simulink model "ControllerTuneLianxi"  (Simulink 9.1)
settings: Solver=VariableStepAuto  StartTime=0.0  StopTime=10  RelTol=1e-3
PreLoadFcn:
  | clear
  | A=[-0.0313 4.4879 0 -9.8; ...
  |    -0.0058 -0.7458 0.9480 0; ...
  |    -0.0002 -0.4479 -0.4609 0; ...
  |    0 0 1 0];
  | B = [0.2063 -0.0516 -0.6532 0; ...
  |      3.4847 -0.0561 0.0193 0]';
  | C = eye(4);
  | D = [0 0 0 0; 0 0 0 0]';
  | Ktheta = 0;
  | KthetaI = 0;
  | KthetaD = 0;
  | Kq = 0;
  | KthetaV = 0;
  | KqV = 0;
  | KDeltaV = 0;
  | Ltheta = 0;
  | Lq = 0;
  | LV = 0;
  | LVI = 0;
  | LVdot = 0;
libraries: simulink x7, checkpacklib x2
settings Model: Creator=McQueen_Zero  LastModifiedBy=McQueen_Zero
settings DataIOCC: SaveFormat=Dataset
settings OptimizationCC: LifeSpan=auto
settings DebuggingCC: UnderspecifiedInitializationDetection=Simplified  MergeDetectMultiDrivingBlocksExec=error  SFUnexpectedBacktrackingDiag=error  SFNoUnconditionalDefaultTransitionDiag=error  SFExecutionAtInitializationDiag=warning
settings HardwareCC: ProdBitPerPointer=64  ProdBitPerSizeT=64  ProdBitPerPtrDiffT=64  ProdLargestAtomicFloat=Float  ProdIntDivRoundTo=Zero  ProdEndianess=LittleEndian  ProdWordSize=64  ProdHWDeviceType=Intel->x86-64 (Windows64)
settings ModelReferenceCC: PropagateSignalLabelsOutOfModel=on
settings CodeAppCC: StateflowObjectComments=off
settings GRTTargetCC: TargetLangStandard=C99 (ISO)  CombineOutputUpdateFcns=on  GRTInterface=off
settings ConfigComp: CovMetricSettings=dwe  CovHtmlReporting=off  CovSaveCumulativeToWorkspaceVar=off  CovSaveSingleToWorkspaceVar=off  CovExternalEMLEnable=on

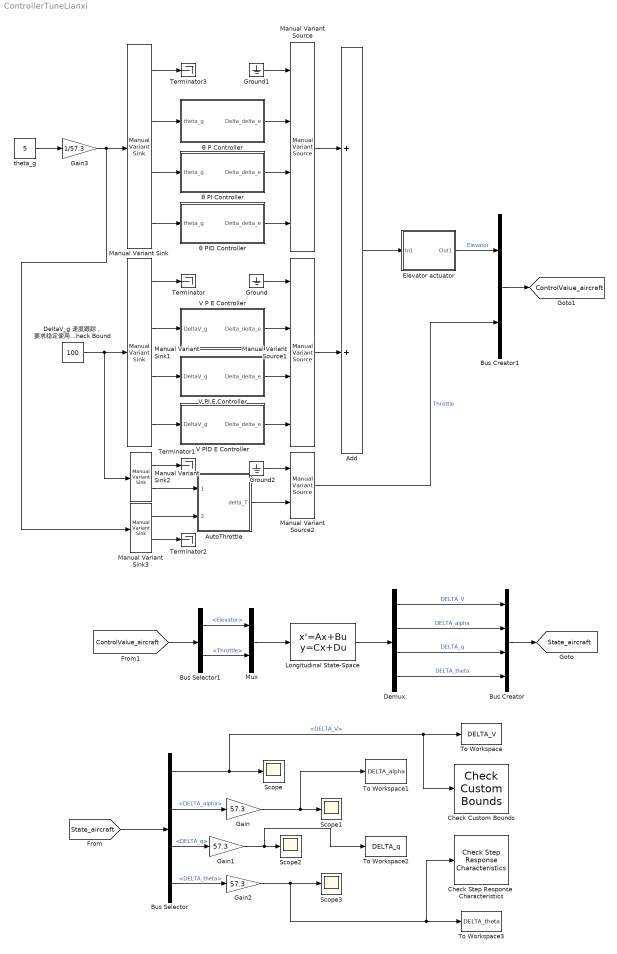
== system ControllerTuneLianxi ==
  Add : Sum
  AutoThrottle : Subsystem  mask{KthetaV=KthetaV, KqV=KqV, KDeltaV=KDeltaV}
      mask prompts: KthetaV "俯仰角增量比例系数"; KqV "俯仰角速率比例系数"; KDeltaV "速度增量比例系数"
  Bus Creator : BusCreator  Inputs=4
  Bus Creator1 : BusCreator  Inputs=2
  Bus Selector : BusSelector  OutputSignals=DELTA_V,DELTA_alpha,DELTA_q,DELTA_theta
  Bus Selector1 : BusSelector  OutputSignals=Elevator,Throttle
  Check Custom Bounds : checkpacklib/Check Custom Bounds  InstantiateOnLoad=on  enabled=on  stopWhenAssertionFail=off  export=off  ViewDlgPos=[]  OpenViewOnLoad=off  LaunchViewOnOpen=off  TimeUnits=seconds  EnableUpperBound=on  UpperBoundTimes=[0 10]  UpperBoundAmplitudes=[1 1]  EnableLowerBound=on  LowerBoundTimes=[0 10]  LowerBoundAmplitudes=[-1 -1]
  Check Step Response  Characteristics : checkpacklib/Check Step Response  Characteristics  InstantiateOnLoad=on  enabled=on  stopWhenAssertionFail=off  export=off  ViewDlgPos=[]  OpenViewOnLoad=off  LaunchViewOnOpen=off  TimeUnits=seconds  EnableStepResponseBound=on  InitialValue=0  FinalValue=5  StepTime=0  RiseTime=2  PercentRise=20  SettlingTime=3  PercentSettling=1  PercentOvershoot=5  PercentUndershoot=1
  "DeltaV_g 速度跟踪， 要求稳定使用 Check Bound " : Constant  Value=100
  Demux : Demux
  Elevator actuator : Subsystem
  Gain : Gain  Gain=57.3
  Gain1 : Gain  Gain=57.3
  Gain2 : Gain  Gain=57.3
  Gain3 : Gain  Gain=1/57.3
  Ground : Ground
  Ground1 : Ground
  Ground2 : Ground
  Longitudinal State-Space : StateSpace  A=A  B=B  C=C  D=D  InitialCondition=0
  Manual Variant Sink : simulink/Signal Routing/Manual Variant Sink  NumChoices=4  OverrideUsingVariant=V_3
      settings: SourceProductName=Simulink
  Manual Variant Sink1 : simulink/Signal Routing/Manual Variant Sink  NumChoices=4  OverrideUsingVariant=V_1
      settings: SourceProductName=Simulink
  Manual Variant Sink2 : simulink/Signal Routing/Manual Variant Sink  NumChoices=2  OverrideUsingVariant=V_1
      settings: SourceProductName=Simulink
  Manual Variant Sink3 : simulink/Signal Routing/Manual Variant Sink  NumChoices=2  OverrideUsingVariant=V_1
      settings: SourceProductName=Simulink
  Manual Variant Source : simulink/Signal Routing/Manual Variant Source  NumChoices=4  OverrideUsingVariant=V_3
      settings: SourceProductName=Simulink
  Manual Variant Source1 : simulink/Signal Routing/Manual Variant Source  NumChoices=4  OverrideUsingVariant=V_1
      settings: SourceProductName=Simulink
  Manual Variant Source2 : simulink/Signal Routing/Manual Variant Source  NumChoices=2  OverrideUsingVariant=V_2
      settings: SourceProductName=Simulink
  Mux : Mux  Inputs=2
  Scope{,1..3} (4 alike) : Scope
  Terminator{,1..3} (4 alike) : Terminator
  To Workspace : ToWorkspace  VariableName=DELTA_V  SaveFormat=Timeseries  SampleTime=-1
  To Workspace1 : ToWorkspace  VariableName=DELTA_alpha  SaveFormat=Timeseries  SampleTime=-1
  To Workspace2 : ToWorkspace  VariableName=DELTA_q  SaveFormat=Timeseries  SampleTime=-1
  To Workspace3 : ToWorkspace  VariableName=DELTA_theta  SaveFormat=Timeseries  SampleTime=-1
  V P E Controller : Subsystem  mask{LV=LV, Ltheta=Ltheta, Lq=Lq}
      mask prompts: LV "速度系数"; Ltheta "俯仰角系数"; Lq "俯仰角速率系数"
  V PI E Controller : Subsystem  mask{LV=LV, LVI=LVI, Ltheta=Ltheta, Lq=Lq}
      mask prompts: LV "速度系数"; LVI "速度积分系数"; Ltheta "俯仰角系数"; Lq "俯仰角速率系数"
  V PID E Controller : Subsystem  mask{LV=LV, LVI=LVI, LVdot=LVdot, Ltheta=Ltheta, Lq=Lq}
      mask prompts: LV "速度系数"; LVI "速度积分系数"; LVdot "速度微分系数"; Ltheta "俯仰角系数"; Lq "俯仰角速率系数"
  theta_g : Constant  Value=5
  θ P Controller : Subsystem  mask{Ktheta=Ktheta, Kq=Kq}
      mask prompts: Ktheta "俯仰角比例系数"; Kq "俯仰角速率比例系数"
  θ PI Controller : Subsystem  mask{Ktheta=Ktheta, KthetaI=KthetaI, Kq=Kq}
      mask prompts: Ktheta "俯仰角比例系数"; KthetaI "俯仰角积分系数"; Kq "俯仰角速率比例系数"
  θ PID Controller : Subsystem  mask{Ktheta=Ktheta, KthetaI=KthetaI, KthetaD=KthetaD, Kq=Kq}
      mask prompts: Ktheta "俯仰角比例系数"; KthetaI "俯仰角积分系数"; KthetaD "俯仰角微分系数"; Kq "俯仰角速率比例系数"
  tag scope: ControlValue_aircraft=global, State_aircraft=global
  wires:
  Demux/3 -> Bus Creator/3  "DELTA_q"
  Gain1/1 -> To Workspace2/1, Scope2/1
  Bus Selector/4 -> Gain2/1  "<DELTA_theta>"
  Bus Selector/2 -> Gain/1  "<DELTA_alpha>"
  Bus Selector/3 -> Gain1/1  "<DELTA_q>"
  [State_aircraft] -> Bus Selector/1
  Demux/2 -> Bus Creator/2  "DELTA_alpha"
  Demux/4 -> Bus Creator/4  "DELTA_theta"
  Demux/1 -> Bus Creator/1  "DELTA_V"
  Gain/1 -> To Workspace1/1, Scope1/1
  Mux/1 -> Longitudinal State-Space/1
  Longitudinal State-Space/1 -> Demux/1
  Bus Creator/1 -> [State_aircraft]
  Gain2/1 -> Check Step Response  Characteristics/1, To Workspace3/1, Scope3/1
  Bus Selector/1 -> Check Custom Bounds/1, To Workspace/1, Scope/1  "<DELTA_V>"
  Bus Selector1/2 -> Mux/2  "<Throttle>"
  Bus Selector1/1 -> Mux/1  "<Elevator>"
  [ControlValue_aircraft] -> Bus Selector1/1
  Elevator actuator/1(Out1) -> Bus Creator1/1  "Elevator"
  Bus Creator1/1 -> [ControlValue_aircraft]
  theta_g/1 -> Gain3/1
  θ P Controller/1(Delta_delta_e) -> Manual Variant Source/2
  θ PI Controller/1(Delta_delta_e) -> Manual Variant Source/3
  θ PID Controller/1(Delta_delta_e) -> Manual Variant Source/4
  Manual Variant Sink/2 -> θ P Controller/1(theta_g)
  Manual Variant Sink/3 -> θ PI Controller/1(theta_g)
  Manual Variant Sink/4 -> θ PID Controller/1(theta_g)
  Gain3/1 -> Manual Variant Sink3/1, Manual Variant Sink/1
  Add/1 -> Elevator actuator/1(In1)
  Manual Variant Source/1 -> Add/1
  V P E Controller/1(Delta_delta_e) -> Manual Variant Source1/2
  Manual Variant Source1/1 -> Add/2
  Ground/1 -> Manual Variant Source1/1
  "DeltaV_g 速度跟踪， 要求稳定使用 Check Bound "/1 -> Manual Variant Sink2/1, Manual Variant Sink1/1
  Manual Variant Sink1/2 -> V P E Controller/1(DeltaV_g)
  Manual Variant Sink1/3 -> V PI E Controller/1(DeltaV_g)
  Manual Variant Sink1/4 -> V PID E Controller/1(DeltaV_g)
  V PI E Controller/1(Delta_delta_e) -> Manual Variant Source1/3
  V PID E Controller/1(Delta_delta_e) -> Manual Variant Source1/4
  Manual Variant Sink1/1 -> Terminator/1
  Manual Variant Sink2/1 -> Terminator1/1
  Manual Variant Sink3/2 -> Terminator2/1
  Manual Variant Sink2/2 -> AutoThrottle/1(DeltaV_g)
  Manual Variant Sink3/1 -> AutoThrottle/2(theta_g)
  Manual Variant Sink/1 -> Terminator3/1
  Ground1/1 -> Manual Variant Source/1
  AutoThrottle/1(delta_T) -> Manual Variant Source2/2
  Ground2/1 -> Manual Variant Source2/1
  Manual Variant Source2/1 -> Bus Creator1/2  "Throttle"

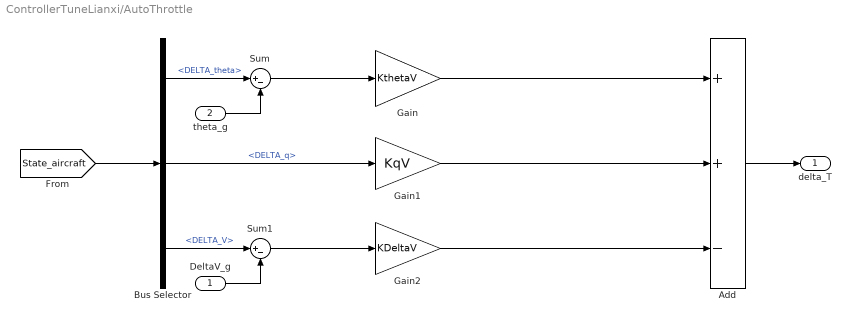
== system ControllerTuneLianxi/AutoThrottle ==
  DeltaV_g : Inport
  theta_g : Inport  Port=2
  Add : Sum  Inputs=++-
  Bus Selector : BusSelector  OutputSignals=DELTA_theta,DELTA_q,DELTA_V
  Gain : Gain  Gain=KthetaV
  Gain1 : Gain  Gain=KqV
  Gain2 : Gain  Gain=KDeltaV
  Sum : Sum  Inputs=|+-
  Sum1 : Sum  Inputs=|+-
  delta_T : Outport
  wires:
  [State_aircraft] -> Bus Selector/1
  Add/1 -> delta_T/1
  Gain1/1 -> Add/2
  Gain/1 -> Add/1
  Bus Selector/2 -> Gain1/1  "<DELTA_q>"
  Bus Selector/1 -> Sum/1  "<DELTA_theta>"
  Bus Selector/3 -> Sum1/1  "<DELTA_V>"
  Sum/1 -> Gain/1
  theta_g/1 -> Sum/2
  Sum1/1 -> Gain2/1
  DeltaV_g/1 -> Sum1/2
  Gain2/1 -> Add/3

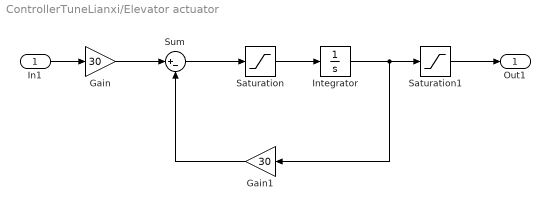
== system ControllerTuneLianxi/Elevator actuator ==
  In1 : Inport
  Gain : Gain  Gain=30
  Gain1 : Gain  Gain=30
  Integrator : Integrator
  Saturation : Saturate  UpperLimit=180  LowerLimit=-180
  Saturation1 : Saturate  UpperLimit=30  LowerLimit=-30
  Sum : Sum  Inputs=|+-
  Out1 : Outport
  wires:
  Saturation/1 -> Integrator/1
  Saturation1/1 -> Out1/1
  In1/1 -> Gain/1
  Gain/1 -> Sum/1
  Sum/1 -> Saturation/1
  Gain1/1 -> Sum/2
  Integrator/1 -> Gain1/1, Saturation1/1

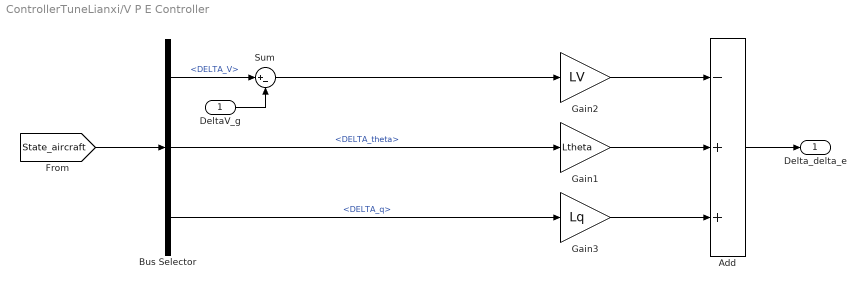
== system ControllerTuneLianxi/V P E Controller ==
  DeltaV_g : Inport
  Add : Sum  Inputs=-++
  Bus Selector : BusSelector  OutputSignals=DELTA_V,DELTA_theta,DELTA_q
  Gain1 : Gain  Gain=Ltheta
  Gain2 : Gain  Gain=LV
  Gain3 : Gain  Gain=Lq
  Sum : Sum  Inputs=|+-
  Delta_delta_e : Outport
  wires:
  [State_aircraft] -> Bus Selector/1
  DeltaV_g/1 -> Sum/2
  Bus Selector/1 -> Sum/1  "<DELTA_V>"
  Sum/1 -> Gain2/1
  Add/1 -> Delta_delta_e/1
  Gain2/1 -> Add/1
  Gain1/1 -> Add/2
  Gain3/1 -> Add/3
  Bus Selector/3 -> Gain3/1  "<DELTA_q>"
  Bus Selector/2 -> Gain1/1  "<DELTA_theta>"

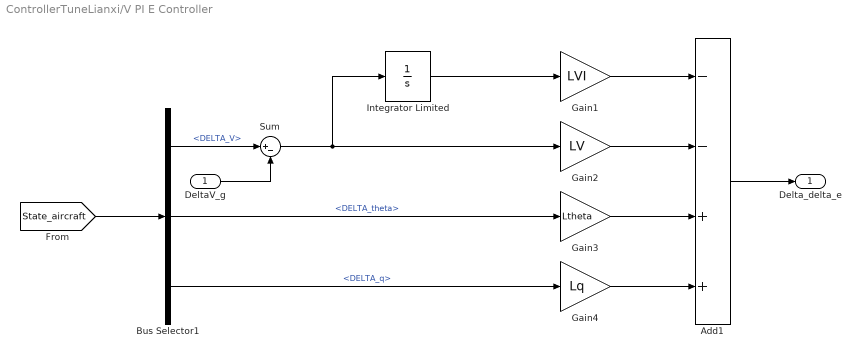
== system ControllerTuneLianxi/V PI E Controller ==
  DeltaV_g : Inport
  Add1 : Sum  Inputs=--++
  Bus Selector1 : BusSelector  OutputSignals=DELTA_V,DELTA_theta,DELTA_q
  Gain1 : Gain  Gain=LVI
  Gain2 : Gain  Gain=LV
  Gain3 : Gain  Gain=Ltheta
  Gain4 : Gain  Gain=Lq
  Integrator Limited : Integrator  LimitOutput=on  UpperSaturationLimit=30/57.3  LowerSaturationLimit=0
  Sum : Sum  Inputs=|+-
  Delta_delta_e : Outport
  wires:
  Add1/1 -> Delta_delta_e/1
  [State_aircraft] -> Bus Selector1/1
  DeltaV_g/1 -> Sum/2
  Bus Selector1/1 -> Sum/1  "<DELTA_V>"
  Gain2/1 -> Add1/2
  Sum/1 -> Integrator Limited/1, Gain2/1
  Gain1/1 -> Add1/1
  Integrator Limited/1 -> Gain1/1
  Gain3/1 -> Add1/3
  Gain4/1 -> Add1/4
  Bus Selector1/3 -> Gain4/1  "<DELTA_q>"
  Bus Selector1/2 -> Gain3/1  "<DELTA_theta>"

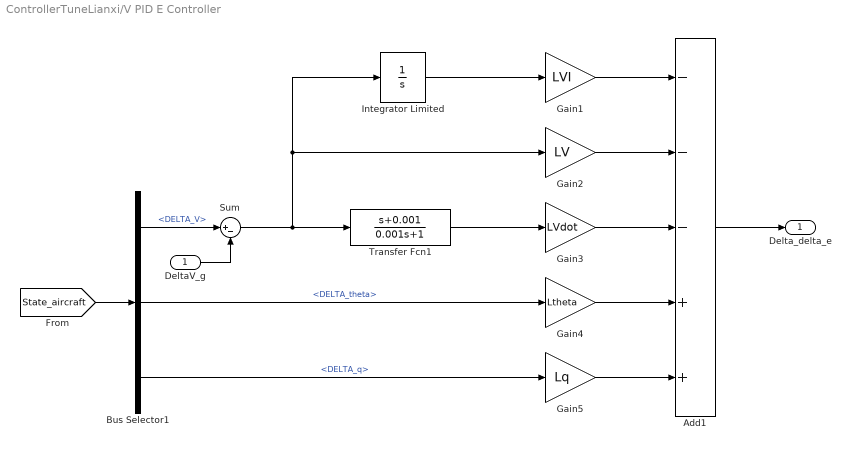
== system ControllerTuneLianxi/V PID E Controller ==
  DeltaV_g : Inport
  Add1 : Sum  Inputs=---++
  Bus Selector1 : BusSelector  OutputSignals=DELTA_V,DELTA_theta,DELTA_q
  Gain1 : Gain  Gain=LVI
  Gain2 : Gain  Gain=LV
  Gain3 : Gain  Gain=LVdot
  Gain4 : Gain  Gain=Ltheta
  Gain5 : Gain  Gain=Lq
  Integrator Limited : Integrator  LimitOutput=on  UpperSaturationLimit=30/57.3  LowerSaturationLimit=0
  Sum : Sum  Inputs=|+-
  Transfer Fcn1 : TransferFcn  Numerator=[1 0.001]  Denominator=[0.001 1]
  Delta_delta_e : Outport
  wires:
  Add1/1 -> Delta_delta_e/1
  [State_aircraft] -> Bus Selector1/1
  DeltaV_g/1 -> Sum/2
  Bus Selector1/1 -> Sum/1  "<DELTA_V>"
  Transfer Fcn1/1 -> Gain3/1
  Gain3/1 -> Add1/3
  Gain2/1 -> Add1/2
  Sum/1 -> Integrator Limited/1, Gain2/1, Transfer Fcn1/1
  Gain1/1 -> Add1/1
  Integrator Limited/1 -> Gain1/1
  Gain4/1 -> Add1/4
  Gain5/1 -> Add1/5
  Bus Selector1/3 -> Gain5/1  "<DELTA_q>"
  Bus Selector1/2 -> Gain4/1  "<DELTA_theta>"

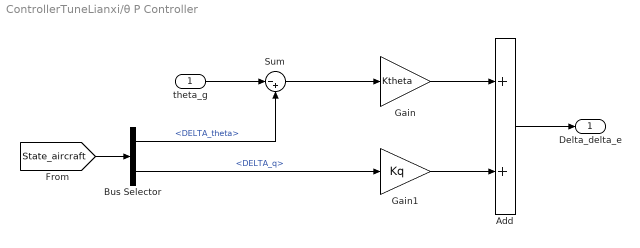
== system ControllerTuneLianxi/θ P Controller ==
  theta_g : Inport
  Add : Sum
  Bus Selector : BusSelector  OutputSignals=DELTA_theta,DELTA_q
  Gain : Gain  Gain=Ktheta
  Gain1 : Gain  Gain=Kq
  Sum : Sum  Inputs=|-+
  Delta_delta_e : Outport
  wires:
  theta_g/1 -> Sum/1
  Add/1 -> Delta_delta_e/1
  Gain/1 -> Add/1
  Sum/1 -> Gain/1
  Gain1/1 -> Add/2
  [State_aircraft] -> Bus Selector/1
  Bus Selector/1 -> Sum/2  "<DELTA_theta>"
  Bus Selector/2 -> Gain1/1  "<DELTA_q>"

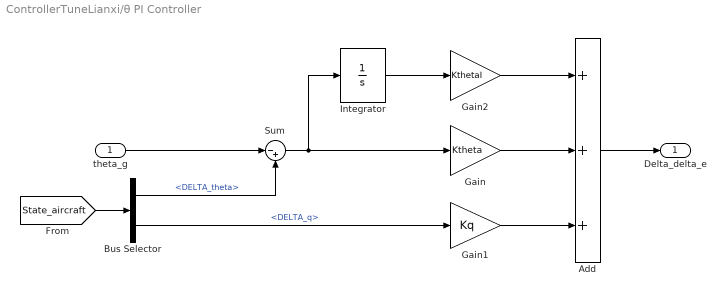
== system ControllerTuneLianxi/θ PI Controller ==
  theta_g : Inport
  Add : Sum  Inputs=+++
  Bus Selector : BusSelector  OutputSignals=DELTA_theta,DELTA_q
  Gain : Gain  Gain=Ktheta
  Gain1 : Gain  Gain=Kq
  Gain2 : Gain  Gain=KthetaI
  Integrator : Integrator  LimitOutput=on  UpperSaturationLimit=30/57.3  LowerSaturationLimit=0
  Sum : Sum  Inputs=|-+
  Delta_delta_e : Outport
  wires:
  theta_g/1 -> Sum/1
  Add/1 -> Delta_delta_e/1
  Gain/1 -> Add/2
  Sum/1 -> Gain/1, Integrator/1
  Gain1/1 -> Add/3
  [State_aircraft] -> Bus Selector/1
  Bus Selector/1 -> Sum/2  "<DELTA_theta>"
  Bus Selector/2 -> Gain1/1  "<DELTA_q>"
  Gain2/1 -> Add/1
  Integrator/1 -> Gain2/1

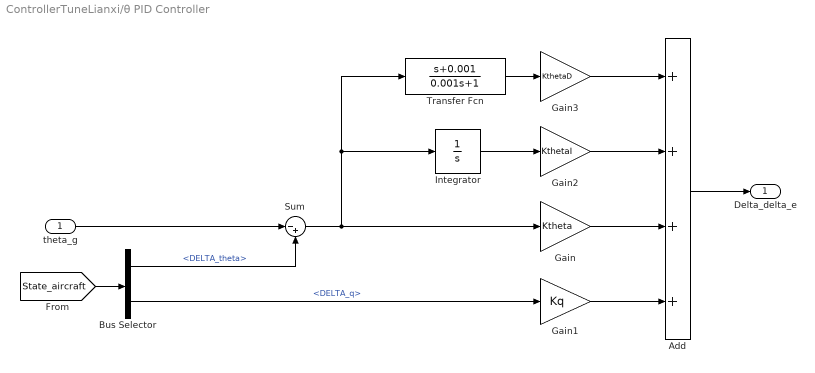
== system ControllerTuneLianxi/θ PID Controller ==
  theta_g : Inport
  Add : Sum  Inputs=++++
  Bus Selector : BusSelector  OutputSignals=DELTA_theta,DELTA_q
  Gain : Gain  Gain=Ktheta
  Gain1 : Gain  Gain=Kq
  Gain2 : Gain  Gain=KthetaI
  Gain3 : Gain  Gain=KthetaD
  Integrator : Integrator  LimitOutput=on  UpperSaturationLimit=30/57.3  LowerSaturationLimit=0
  Sum : Sum  Inputs=|-+
  Transfer Fcn : TransferFcn  Numerator=[1 0.001]  Denominator=[0.001 1]
  Delta_delta_e : Outport
  wires:
  theta_g/1 -> Sum/1
  Add/1 -> Delta_delta_e/1
  Gain/1 -> Add/3
  Sum/1 -> Integrator/1, Transfer Fcn/1, Gain/1
  Gain1/1 -> Add/4
  [State_aircraft] -> Bus Selector/1
  Bus Selector/1 -> Sum/2  "<DELTA_theta>"
  Bus Selector/2 -> Gain1/1  "<DELTA_q>"
  Gain2/1 -> Add/2
  Integrator/1 -> Gain2/1
  Gain3/1 -> Add/1
  Transfer Fcn/1 -> Gain3/1
